simulink library "Cassie_CommandBlock_Library_5"  (R2017b)
settings: Solver=VariableStepAuto  StartTime=0.0  StopTime=10.0  RelTol=1e-3
undefined symbols (not defined in the file): dq, DynamicMatrixLibrary, isSim, q, sample_time
libraries: slrtlib x125, Cassie_CommandBlock_Library_3 x1
(part 3 of 3)

== matlab function Cassie_CommandBlock_Library_5/Subsystem/MATLAB Function ==
  data: dq input; dqxyz input; dq output; EulerRates input
function dq = mix_dq(dq,dqxyz,EulerRates)
dq(1:3) = dqxyz;
dq(4:6) = EulerRates;
